simulink model "rlSimplePendulumModel_bus"  (R2020a)
settings: Solver=ode45  StartTime=0.0  StopTime=Tf  RelTol=1e-5  AbsTol=1e-6
model workspace (MAT data in the model file):
  I = 0
  c = 0
  g = 9.81
  l = 1
  m = 1
  max_tau = 2
  theta0 = 0
  theta_dot0 = 0
libraries: rllib x1
settings Model: Creator=The MathWorks, Inc.  LastModifiedBy=The MathWorks, Inc.
settings SolverCC: AutoScaleAbsTol=off
settings DataIOCC: LimitDataPoints=on  SaveFormat=Array  SaveState=on
settings OptimizationCC: BlockReduction=off  BooleanDataType=off  LifeSpan=inf
settings DebuggingCC: SaveWithParameterizedLinksMsg=none  SignalResolutionControl=TryResolveAllWithWarning  SFUnexpectedBacktrackingDiag=warning  SFNoUnconditionalDefaultTransitionDiag=warning  SFExecutionAtInitializationDiag=none  ArithmeticOperatorsInVariantConditions=warning
settings HardwareCC: ProdBitPerPointer=32  ProdBitPerSizeT=32  ProdBitPerPtrDiffT=32  ProdLargestAtomicFloat=None  ProdIntDivRoundTo=Undefined  ProdEndianess=Unspecified  ProdWordSize=32  ProdHWDeviceType=32-bit Generic  TargetUnknown=on
settings ModelReferenceCC: PropagateSignalLabelsOutOfModel=off
settings SFSimCC: SimUseLocalCustomCode=off  CustomCodeUndefinedFunction=UseInterfaceOnly
settings RTWCC: RTWUseLocalCustomCode=off
settings CodeAppCC: StateflowObjectComments=on
settings GRTTargetCC: TargetLangStandard=C89/C90 (ANSI)
settings ConfigComp: CovMetricSettings=dw  CovHtmlReporting=on  CovSaveCumulativeToWorkspaceVar=on  CovSaveSingleToWorkspaceVar=on  CovExternalEMLEnable=off

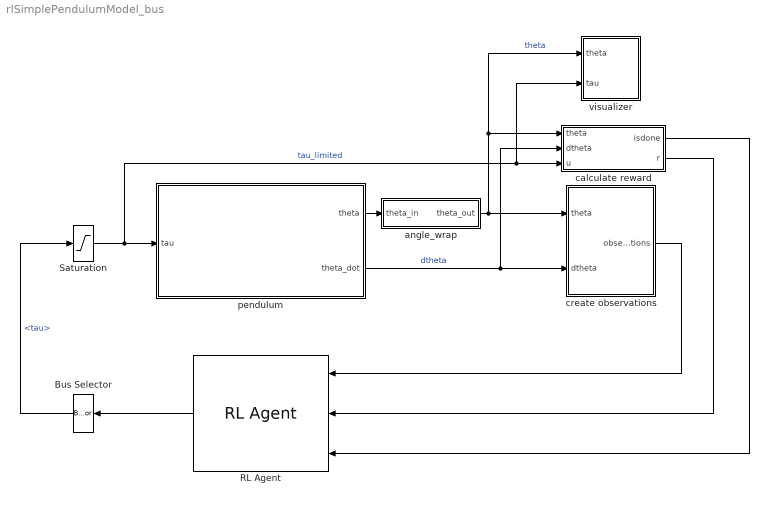
== system rlSimplePendulumModel_bus ==
  Bus Selector : BusSelector  OutputSignals=tau
  RL Agent : rllib/RL Agent  Agent=agent  ProvideReward=on  ProvideIsDone=on  ProvideCumRwd=off  TreatAsDirectFeedthrough=on  CollectLoggedSignals=on  CollectModelStates=on
  Saturation : Saturate  UpperLimit=max_tau  LowerLimit=-max_tau
  angle_wrap : Subsystem
  calculate reward : Subsystem
  create observations : Subsystem  VariantControl=sincos
  pendulum : Subsystem
  visualizer : Subsystem
  wires:
  pendulum/2(theta_dot) -> create observations/2(dtheta), calculate reward/2(dtheta)  "dtheta"
  pendulum/1(theta) -> angle_wrap/1(theta_in)
  angle_wrap/1(theta_out) -> create observations/1(theta), visualizer/1(theta), calculate reward/1(theta)  "theta"
  calculate reward/2(r) -> RL Agent/2
  calculate reward/1(isdone) -> RL Agent/3
  Saturation/1 -> visualizer/2(tau), calculate reward/3(u), pendulum/1(tau)  "tau_limited"
  create observations/1(observations) -> RL Agent/1
  RL Agent/1 -> Bus Selector/1
  Bus Selector/1 -> Saturation/1  "<tau>"

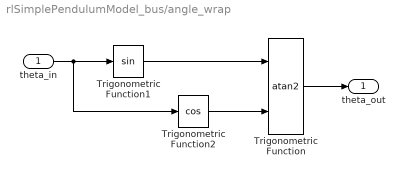
== system rlSimplePendulumModel_bus/angle_wrap ==
  theta_in : Inport
  Trigonometric Function : Trigonometry  Operator=atan2
  Trigonometric Function1 : Trigonometry
  Trigonometric Function2 : Trigonometry  Operator=cos
  theta_out : Outport  VectorParamsAs1DForOutWhenUnconnected=off
  wires:
  theta_in/1 -> Trigonometric Function2/1, Trigonometric Function1/1
  Trigonometric Function/1 -> theta_out/1
  Trigonometric Function1/1 -> Trigonometric Function/1
  Trigonometric Function2/1 -> Trigonometric Function/2

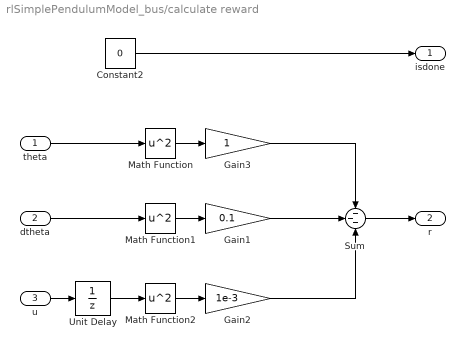
== system rlSimplePendulumModel_bus/calculate reward ==
  theta : Inport
  dtheta : Inport  Port=2
  u : Inport  Port=3
  Constant2 : Constant  Value=0
  Gain1 : Gain  Gain=0.1
  Gain2 : Gain  Gain=1e-3
  Gain3 : Gain
  Math Function : Math  Operator=square  SignedPower=on  SaturateOnIntegerOverflow=on
  Math Function1 : Math  Operator=square  SignedPower=on  SaturateOnIntegerOverflow=on
  Math Function2 : Math  Operator=square  SignedPower=on  SaturateOnIntegerOverflow=on
  Sum : Sum  Inputs=---
  Unit Delay : UnitDelay  SampleTime=-1  HasFrameUpgradeWarning=on
  isdone : Outport  VectorParamsAs1DForOutWhenUnconnected=off
  r : Outport  Port=2  VectorParamsAs1DForOutWhenUnconnected=off
  wires:
  Constant2/1 -> isdone/1
  theta/1 -> Math Function/1
  dtheta/1 -> Math Function1/1
  u/1 -> Unit Delay/1
  Sum/1 -> r/1
  Math Function/1 -> Gain3/1
  Math Function1/1 -> Gain1/1
  Math Function2/1 -> Gain2/1
  Gain2/1 -> Sum/3
  Gain1/1 -> Sum/2
  Gain3/1 -> Sum/1
  Unit Delay/1 -> Math Function2/1

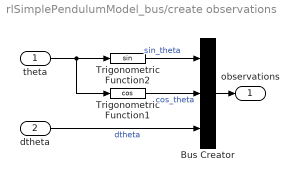
== system rlSimplePendulumModel_bus/create observations ==
  theta : Inport
  dtheta : Inport  Port=2
  Bus Creator : BusCreator  Inputs=3  OutDataTypeStr=Bus: obsBus  NonVirtualBus=on
  Trigonometric Function1 : Trigonometry  Operator=cos
  Trigonometric Function2 : Trigonometry
  observations : Outport  VectorParamsAs1DForOutWhenUnconnected=off
  wires:
  theta/1 -> Trigonometric Function1/1, Trigonometric Function2/1
  Bus Creator/1 -> observations/1
  dtheta/1 -> Bus Creator/3  "dtheta"
  Trigonometric Function2/1 -> Bus Creator/1  "sin_theta"
  Trigonometric Function1/1 -> Bus Creator/2  "cos_theta"

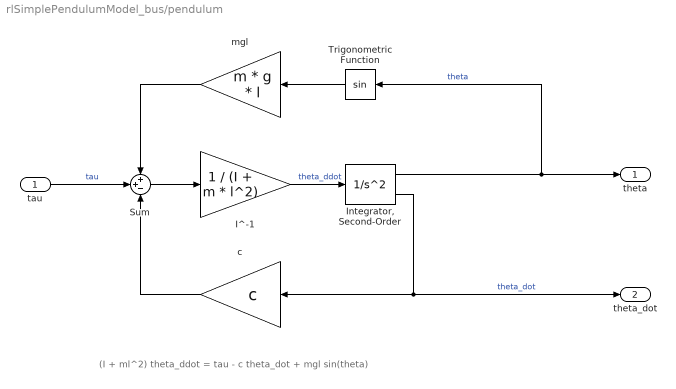
== system rlSimplePendulumModel_bus/pendulum ==
  note: (I + ml^2) theta_ddot = tau - c theta_dot + mgl sin(theta)
  tau : Inport
  I^-1 : Gain  Gain=1 / (I + m * l^2)
  "Integrator, Second-Order" : SecondOrderIntegrator  ICX=theta0  UpperLimitX=1  LowerLimitX=0  StateNameX='theta'  ICDXDT=theta_dot0  StateNameDXDT='theta_dot'
  Sum : Sum  Inputs=++-
  Trigonometric Function : Trigonometry
  c : Gain  Gain=c
  mgl : Gain  Gain=m * g * l
  theta : Outport  VectorParamsAs1DForOutWhenUnconnected=off
  theta_dot : Outport  Port=2  VectorParamsAs1DForOutWhenUnconnected=off
  wires:
  mgl/1 -> Sum/1
  c/1 -> Sum/3
  Trigonometric Function/1 -> mgl/1
  Sum/1 -> I^-1/1
  "Integrator, Second-Order"/1 -> theta/1, Trigonometric Function/1  "theta"
  I^-1/1 -> "Integrator, Second-Order"/1  "theta_ddot"
  "Integrator, Second-Order"/2 -> c/1, theta_dot/1  "theta_dot"
  tau/1 -> Sum/2  "tau"

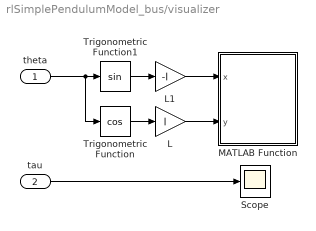
== system rlSimplePendulumModel_bus/visualizer ==
  theta : Inport
  tau : Inport  Port=2
  L : Gain  Gain=l
  L1 : Gain  Gain=-l
  MATLAB Function : MATLAB Function  TreatAsAtomicUnit=on
  Scope : Scope
  Trigonometric Function : Trigonometry  Operator=cos
  Trigonometric Function1 : Trigonometry
  wires:
  tau/1 -> Scope/1
  Trigonometric Function1/1 -> L1/1
  L/1 -> MATLAB Function/2(y)
  Trigonometric Function/1 -> L/1
  L1/1 -> MATLAB Function/1(x)
  theta/1 -> Trigonometric Function1/1, Trigonometric Function/1

== matlab function rlSimplePendulumModel_bus/visualizer/MATLAB Function ==
  settings: updateMethod=DISCRETE
  data: x input; y input
function plotPend(x,y)
% plot the simple pendulum
coder.extrinsic('rl.env.viz.plotSimplePendulum');
rl.env.viz.plotSimplePendulum(x,y);
